simulink model "Altitude_estimation_kalman_filter"  (R2024b)
settings: Solver=VariableStepAuto  StartTime=0.0  StopTime=50  RelTol=1e-3
undefined symbols (not defined in the file): Continuous, Time
libraries: ctrlSharedLib x1

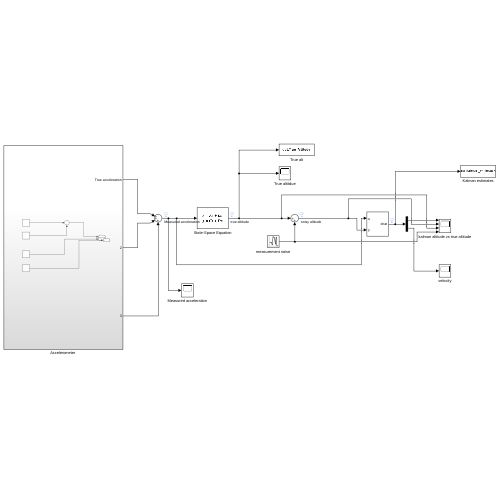
[thumbnail: Simulink's stored preview of the top-level diagram]
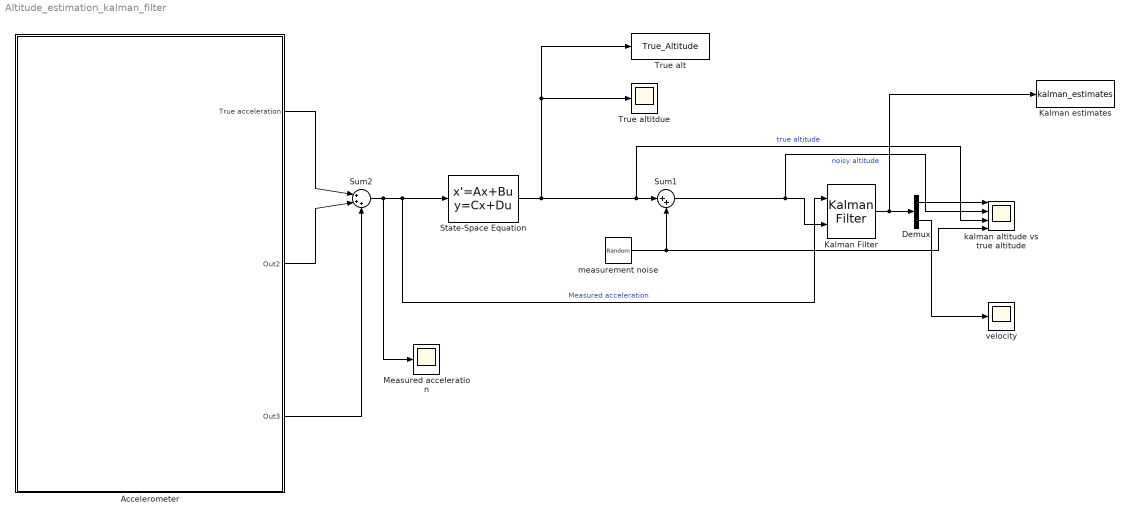
== system Altitude_estimation_kalman_filter ==
  "Accelerometer " : Subsystem
  Demux : Demux  Outputs=2
  Kalman Filter : ctrlSharedLib/Kalman Filter  TimeDomain=Continuous-Time  UseCurrentEstimator=on  ModelSource=Individual A, B, C, D matrices  ModelSourceVariable=ss(0.95,1,1,0,1)  A=[ 0 1; 0 0]  B=[0 ; 1 ]  C=[ 1 0]  D=0  NumberOfStates=1  NumberOfInputs=1  NumberOfOutputs=1  InitialEstimateSource=Dialog  X0=0  P0=10  UseK=off  UseGH=off  NumberOfProcessNoiseInputs=1  G=1  TimeInvariantG=on  H=0  TimeInvariantH=on  Q=[ 0.01 0; 0 1]  TimeInvariantQ=on  R=0.05  TimeInvariantR=on  N=0  TimeInvariantN=on  AddInputPort=on  AddEnablePort=off  OutputEstimatedY=off  OutputP=off  Ts=0.1
  Kalman estimates : ToWorkspace  VariableName=kalman_estimates  SaveFormat=Timeseries  SampleTime=-1
  Measured acceleration : Scope
  State-Space Equation : StateSpace  A=[ 0 1; 0 0]  B=[ 0 ; 1]  C=[ 1 0 ]  D=0  InitialCondition=0
  Sum1 : Sum  Inputs=|++
  Sum2 : Sum  Inputs=|+++
  True alt : ToWorkspace  VariableName=True_Altitude  SaveFormat=Timeseries  SampleTime=-1
  True altitdue : Scope
  kalman altitude vs true altitude : Scope  NumInputPorts=4
  measurement noise : RandomNumber  Variance=0.05  SampleTime=0.1
  velocity : Scope
  wires:
  State-Space Equation/1 -> True alt/1, True altitdue/1, kalman altitude vs true altitude/3, Sum1/1  "true altitude"
  measurement noise/1 -> kalman altitude vs true altitude/4, Sum1/2
  Kalman Filter/1 -> Kalman estimates/1, Demux/1
  Sum1/1 -> kalman altitude vs true altitude/2, Kalman Filter/2  "noisy altitude"
  Demux/2 -> velocity/1
  Sum2/1 -> Measured acceleration/1, Kalman Filter/1, State-Space Equation/1  "Measured acceleration"
  Demux/1 -> kalman altitude vs true altitude/1
  "Accelerometer "/1(True acceleration) -> Sum2/1
  "Accelerometer "/2(Out2) -> Sum2/2
  "Accelerometer "/3(Out3) -> Sum2/3

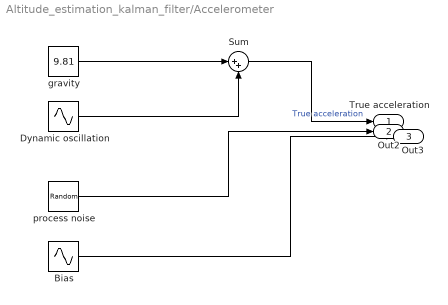
== system Altitude_estimation_kalman_filter/Accelerometer  ==
  Bias : Sin  Amplitude=0.02  Frequency=0.01
  Dynamic oscillation : Sin  Amplitude=0.2  Frequency=0.628
  Sum : Sum  Inputs=|++
  gravity : Constant  Value=9.81
  process noise : RandomNumber  Variance=0.01  SampleTime=0.1
  True acceleration : Outport
  Out2 : Outport  Port=2
  Out3 : Outport  Port=3
  wires:
  Dynamic oscillation/1 -> Sum/2
  Sum/1 -> True acceleration/1  "True acceleration"
  gravity/1 -> Sum/1
  Bias/1 -> Out3/1
  process noise/1 -> Out2/1
